simulink model "traction_control"  (R2019b)
settings: Solver=VariableStepAuto  StartTime=0.0  StopTime=10.0  RelTol=1e-3
libraries: sharedTrackingLibrary x1
settings Model: Creator=michele  LastModifiedBy=michele
settings OptimizationCC: DefaultParameterBehavior=Inlined  EnhancedBackFolding=on  PassReuseOutputArgsAs=Individual arguments  ZeroExternalMemoryAtStartup=off  ZeroInternalMemoryAtStartup=off  OptimizeBlockOrder=speed  DifferentSizesBufferReuse=on  OptimizationCustomize=off  EfficientTunableParamExpr=on
settings DebuggingCC: ParameterTunabilityLossMsg=error
settings SFSimCC: MATLABDynamicMemAlloc=off
settings RTWCC: SystemTargetFile=ert.tlc  TemplateMakefile=ert_default_tmf  GenerateReport=on  IncludeHyperlinkInReport=on  LaunchReport=on  GenerateTraceInfo=on  GenerateTraceReport=on  GenerateTraceReportSl=on  GenerateTraceReportSf=on  GenerateTraceReportEml=on
settings CodeAppCC: ForceParamTrailComments=on  IgnoreCustomStorageClasses=off  OperatorAnnotations=on  SimulinkDataObjDesc=on  SFDataObjDesc=on  InsertBlockDesc=on
settings ERTTargetCC: TargetLangStandard=C99 (ISO)  GenerateSampleERTMain=on  InlinedParameterPlacement=NonHierarchical  ERTCustomFileTemplate=example_file_process.tlc

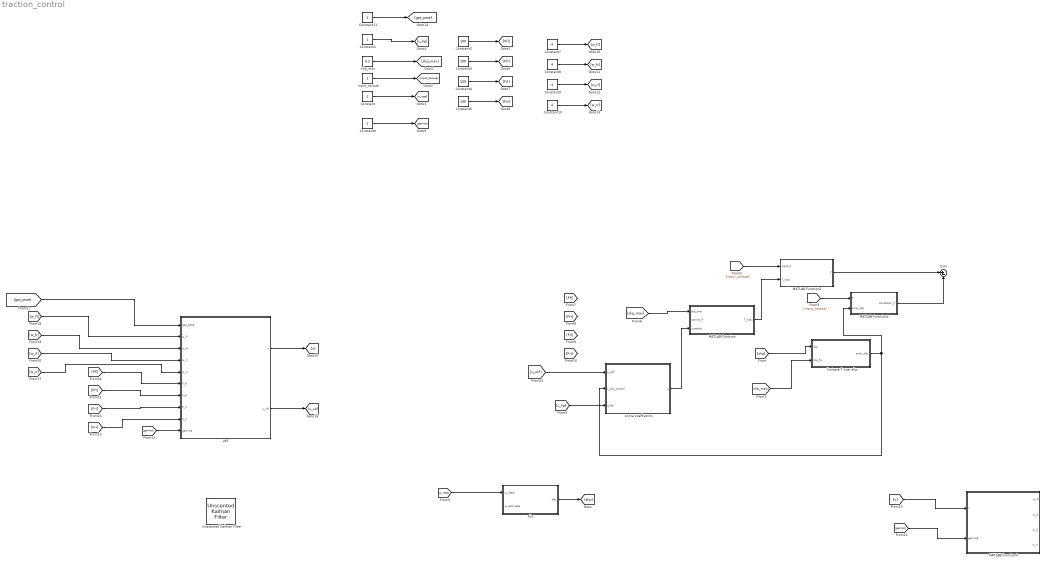
== system traction_control ==
  Constant{,1,6,11} (4 alike) : Constant
  Constant{7..10} (4 alike) : Constant  Value=4
  Constant{2..5} (4 alike) : Constant  Value=100
  MATLAB Function : MATLAB Function  TreatAsAtomicUnit=on
  MATLAB Function1 : MATLAB Function  TreatAsAtomicUnit=on
  MATLAB Function2 : MATLAB Function  TreatAsAtomicUnit=on
  MATLAB Function4 : MATLAB Function  TreatAsAtomicUnit=on
  Sum : Sum  Inputs=|+-
  UKF : MATLAB Function  TreatAsAtomicUnit=on
  Unscented Kalman Filter : sharedTrackingLibrary/Unscented Kalman Filter  StateTransitionFcn=myStateTransitionFcn  HasAdditiveProcessNoise=Additive  ProcessNoise=1  HasTimeVaryingProcessNoise=off  HasStateTransitionFcnExtraArgument=0  InitialState=0  InitialStateCovariance=1  Alpha=1e-3  Beta=2  Kappa=0  MeasurementFcn1=myMeasurementFcn  HasMeasurementEnablePort1=off  HasAdditiveMeasurementNoise1=Additive  MeasurementNoise1=1  HasTimeVaryingMeasurementNoise1=off  HasMeasurementFcnExtraArgument1=0  MeasurementFcn2=myMeasurementFcn  HasMeasurementEnablePort2=off  HasAdditiveMeasurementNoise2=Additive  MeasurementNoise2=1  HasTimeVaryingMeasurementNoise2=off  HasMeasurementFcnExtraArgument2=0  MeasurementFcn3=myMeasurementFcn  HasMeasurementEnablePort3=off  HasAdditiveMeasurementNoise3=Additive  MeasurementNoise3=1  HasTimeVaryingMeasurementNoise3=off  HasMeasurementFcnExtraArgument3=0  MeasurementFcn4=myMeasurementFcn  HasMeasurementEnablePort4=off  HasAdditiveMeasurementNoise4=Additive  MeasurementNoise4=1  HasTimeVaryingMeasurementNoise4=off  HasMeasurementFcnExtraArgument4=0  MeasurementFcn5=myMeasurementFcn  HasMeasurementEnablePort5=off  HasAdditiveMeasurementNoise5=Additive  MeasurementNoise5=1  HasTimeVaryingMeasurementNoise5=off  HasMeasurementFcnExtraArgument5=0  EnableMultirate=off  StateTransitionFcnSampleTime=1  MeasurementFcn1SampleTime=1  MeasurementFcn2SampleTime=1  MeasurementFcn3SampleTime=1  MeasurementFcn4SampleTime=1  MeasurementFcn5SampleTime=1  UseCurrentEstimator=on  OutputStateCovariance=off  DataType=double  SampleTime=1  NumberOfMeasurements=1
      settings: SourceProductName=Automated Driving Toolbox  SourceProductBaseCode=DR
  "input_torque " : Constant
  "limitate T over slip " : MATLAB Function  TreatAsAtomicUnit=on
  "slip " : MATLAB Function  TreatAsAtomicUnit=on
  "slip_max " : Constant  Value=0.2
  stima coeff atrito : MATLAB Function  TreatAsAtomicUnit=on
  wires:
  MATLAB Function/1(T_max) -> MATLAB Function1/2(T_max)
  stima coeff atrito/1(u) -> MATLAB Function/3(u_attrito)
  MATLAB Function1/1(T) -> Sum/1
  "slip "/1(slip) -> [slip]
  [slip] -> "limitate T over slip "/1(slip)
  [slip_max] -> "limitate T over slip "/2(slip_fix)
  [input_torque] -> MATLAB Function1/1(input_T)
  [u_hp] -> stima coeff atrito/3(u_hp)
  [w_read] -> "slip "/1(w_read)
  "limitate T over slip "/1(error_slip) -> MATLAB Function2/2(error_slip), stima coeff atrito/2(u_slip_control)
  MATLAB Function2/1(correction_T) -> Sum/2
  [slip_max] -> MATLAB Function/1(slip_max)
  Constant1/1 -> [u_hp]
  Constant2/1 -> [Ffl]
  Constant3/1 -> [Ffr]
  Constant4/1 -> [Frl]
  Constant5/1 -> [Frr]
  "slip_max "/1 -> [slip_max]
  "input_torque "/1 -> [input_torque]
  Constant/1 -> [w_read]
  Constant6/1 -> [gamma]
  [gamma] -> UKF/10(gamma)
  [Ffl] -> UKF/6(F_fl)
  [Ffr] -> UKF/7(F_fr)
  [Frl] -> UKF/8(F_rl)
  [Frr] -> UKF/9(F_rr)
  Constant8/1 -> [w_fr]
  Constant7/1 -> [w_fl]
  Constant10/1 -> [w_rr]
  Constant9/1 -> [w_rl]
  [w_fr] -> UKF/3(w_fr)
  [w_rr] -> UKF/5(w_rr)
  [w_rl] -> UKF/4(w_rl)
  [w_fl] -> UKF/2(w_fl)
  Constant11/1 -> [gps_pose]
  [gps_pose] -> UKF/1(gps_pose)
  UKF/1(v) -> [v]
  UKF/2(u_ukf) -> [u_ukf]
  [u_ukf] -> stima coeff atrito/1(u_ukf)
  [input_torque] -> MATLAB Function2/1(T)
  [gamma] -> MATLAB Function4/2(gamma)
  [v] -> MATLAB Function4/1(v)

== matlab function traction_control/MATLAB Function1 ==
  data: input_T input; T output; T_max input
function T = bound(input_T,T_max)

T = min(input_t,T_max);

== matlab function traction_control/MATLAB Function ==
  data: slip_max input; T_max output; normal_F input; u_attrito input
function T_max = max_torque(slip_max, normal_F,u_attrito)
%funzione per determinare la massima coppia da applicare senza andare in
%overslip
T_max = slip_max+normal_F+u_attrito;

== matlab function traction_control/stima coeff atrito ==
  data: u_ukf input; u output; u_slip_control input; u_hp input
function u = estimation_u(u_ukf,u_slip_control,u_hp)

u = (u_ukf+u_slip_control+u_hp)/3;

== matlab function traction_control/slip  ==
  data: w_read input; slip output; w_estimate input
function slip = fcn(w_read,w_estimate)

slip = (w_read-w_estimate)/w_estimate;

== matlab function traction_control/limitate T over slip  ==
  data: slip input; error_slip output; slip_fix input
function error_slip = fcn(slip,slip_fix)
if slip<slip_fix
    error_slip=0;
    %add increase in caso di sottostima di u
else
    error_slip=(slip-slip_fix)/slip_fix;

== matlab function traction_control/MATLAB Function2 ==
  data: T input; error_slip input; correction_T output
function correction_T = fcn(T,error_slip)

correction_T = error_slip*T;

== matlab function traction_control/UKF ==
  data: gps_pose input; v output; w_fl input; w_fr input; w_rl input; w_rr input; F_fl input; F_fr input; F_rl input; F_rr input; gamma input; u_ukf output
function [v,u_ukf] = UKF(gps_pose,w_fl,w_fr,w_rl,w_rr,F_fl,F_fr,F_rl,F_rr,gamma)









u_ukf=1;

== matlab function traction_control/MATLAB Function4 ==
  data: v input; w_fl output; gamma input; w_fr output; w_rl output; w_rr output
function [w_fl,w_fr,w_rl,w_rr] = differential(v,gamma)

L=3;%lunghezza veicolo
d_r=0.3;%distanza dall'asse a destra
d_l=0.3;%distanza dall'asse a sinistra
r_wheel=0.02;%raggio ruota

d=L/tan(gamma);
w_cir=v/d;
v=[sqrt((d-d_l)^2+L^2),sqrt((d+d_r)^2+L^2),d-d_l,d+d_r]*w_cir;
w=v*r_wheel;
w_fl=w(1);
w_fr=w(2);
w_rl=w(3);
w_rr=w(4);
